simulink model "motor1"  (R2022b)
settings: Solver=ode3  StartTime=0.0  StopTime=10  FixedStep=0.001  MaxStep=0.0001  RelTol=1e-3
undefined symbols (not defined in the file or in its folder): awu, dac, degs2rpm, diff, National_Instruments, PCIe, pid, rpm2rads, sens, step
libraries: sldrtlib x3
settings Model: SimulationMode=external  ExtModeTrigDuration=50000  Creator=loren  LastModifiedBy=francesch2
settings DataIOCC: ReturnWorkspaceOutputs=off
settings HardwareCC: ProdBitPerLong=64  ProdHWDeviceType=Intel->x86-64 (Linux 64)
settings ModelReferenceCC: EnableRefExpFcnMdlSchedulingChecks=on
settings RTWCC: Description=Simulink Desktop Real-Time  SystemTargetFile=sldrt.tlc  TemplateMakefile=sldrt.tmf  RTWCompilerOptimization=on
settings CodeAppCC: MaxIdLength=95
settings SimulinkDesktopRealTimeCC: TargetLibSuffix=_sldrt.a  TargetPreCompLibLocation=C:\Program Files\MATLAB\R2022b\toolbox\sldrt\lib\win64

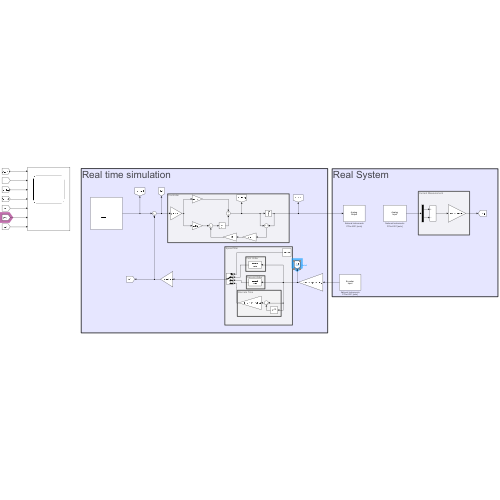
[thumbnail: Simulink's stored preview of the top-level diagram]
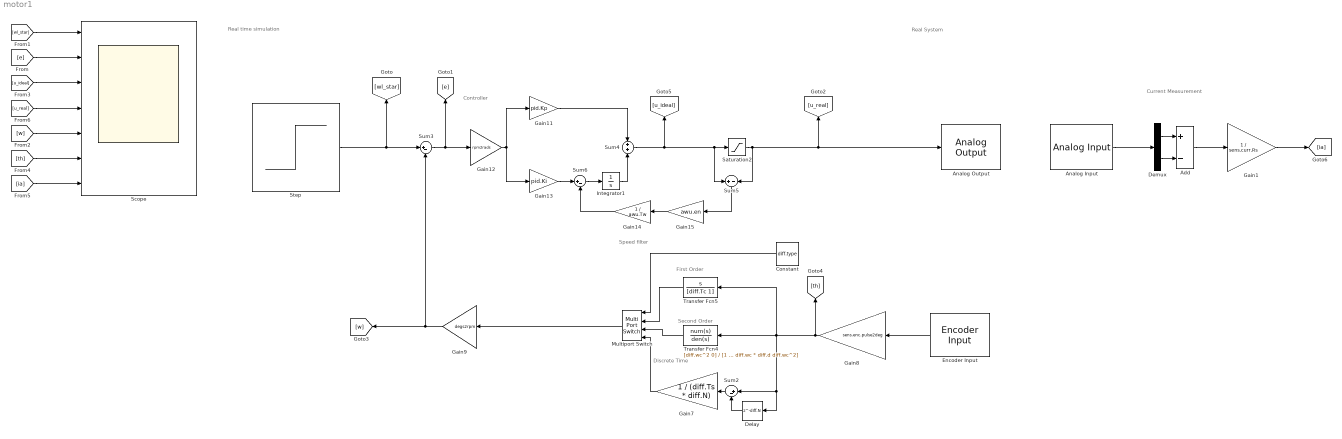
== system motor1 ==
  note: Real time simulation
  note: Controller
  note: Speed filter
  note: Discrete Time
  note: Second Order
  note: First Order
  note: Real System
  note: Current Measurement
  Add : Sum  Inputs=+-
  Analog Input : sldrtlib/Analog Input  SampleTime=-1  MaxMissedTicks=10  ShowMissedTicks=off  YieldWhenWaiting=off  DrvName=National_Instruments/PCIe-6321  DrvAddress=4294967295  DrvOptions=[0 0 0 2 0 0 0]  Channels=[1 2]  RangeMode=1  VoltRange=1  DataType=1
      settings: AttributesFormatString=National Instruments\nPCIe-6321 [auto]
  Analog Output : sldrtlib/Analog Output  SampleTime=-1  MaxMissedTicks=10  ShowMissedTicks=off  YieldWhenWaiting=off  DrvName=National_Instruments/PCIe-6321  DrvAddress=4294967295  DrvOptions=[0 0 0 2 0 0 0]  Channels=1  RangeMode=1  VoltRange=1  InitialValue=0  FinalValue=0
      settings: AttributesFormatString=National Instruments\nPCIe-6321 [auto]
  Constant : Constant  Value=diff.type
  Delay : Delay  DelayLength=diff.N
  Demux : Demux  Outputs=2
  Encoder Input : sldrtlib/Encoder Input  SampleTime=-1  MaxMissedTicks=10  ShowMissedTicks=off  YieldWhenWaiting=off  DrvName=National_Instruments/PCIe-6321  DrvAddress=4294967295  DrvOptions=[0 0 0 2 0 0 0]  Channels=1  QuadMode=3  IndexPulse=1  InputFilter=Inf  DataType=1
      settings: AttributesFormatString=National Instruments\nPCIe-6321 [auto]
  Gain1 : Gain  Gain=1 / sens.curr.Rs
  Gain11 : Gain  Gain=pid.Kp
  Gain12 : Gain  Gain=rpm2rads
  Gain13 : Gain  Gain=pid.Ki
  Gain14 : Gain  Gain=1 / awu.Tw
  Gain15 : Gain  Gain=awu.en
  Gain7 : Gain  Gain=1 / (diff.Ts * diff.N)
  Gain8 : Gain  Gain=sens.enc.pulse2deg
  Gain9 : Gain  Gain=degs2rpm
  Integrator1 : Integrator
  Multiport Switch : MultiPortSwitch  SaturateOnIntegerOverflow=off  InputSameDT=off
  Saturation2 : Saturate  UpperLimit=dac.V  LowerLimit=-dac.V
  Scope : Scope  NumInputPorts=7
  Step : Step  Time=step.T  After=step.A  SampleTime=0
  Sum2 : Sum  Inputs=|+-
  Sum3 : Sum  Inputs=|+-
  Sum4 : Sum  Inputs=+|+
  Sum5 : Sum  Inputs=+|-
  Sum6 : Sum  Inputs=|+-
  Transfer Fcn4 : TransferFcn  Numerator=[diff.wc^2 0]  Denominator=[1 2 * diff.wc * diff.d diff.wc^2]
  Transfer Fcn5 : TransferFcn  Numerator=[1 0]  Denominator=[diff.Tc 1]
  wires:
  Gain8/1 -> Transfer Fcn5/1, Transfer Fcn4/1, Delay/1, Sum2/1, [th]
  Delay/1 -> Sum2/2
  Sum2/1 -> Gain7/1
  Multiport Switch/1 -> Gain9/1
  Transfer Fcn5/1 -> Multiport Switch/2
  Transfer Fcn4/1 -> Multiport Switch/3
  Constant/1 -> Multiport Switch/1
  Gain9/1 -> [w], Sum3/2
  Sum3/1 -> [e], Gain12/1
  Gain12/1 -> Gain11/1, Gain13/1
  Sum4/1 -> Saturation2/1, Sum5/1, [u_ideal]
  Gain11/1 -> Sum4/1
  Integrator1/1 -> Sum4/2
  Gain7/1 -> Multiport Switch/4
  Step/1 -> [wl_star], Sum3/1
  Gain13/1 -> Sum6/1
  Sum6/1 -> Integrator1/1
  Saturation2/1 -> [u_real], Analog Output/1, Sum5/2
  Sum5/1 -> Gain15/1
  Gain14/1 -> Sum6/2
  Gain15/1 -> Gain14/1
  [w] -> Scope/5
  [ia] -> Scope/7
  [wl_star] -> Scope/1
  [u_ideal] -> Scope/3
  [e] -> Scope/2
  Add/1 -> Gain1/1
  Demux/2 -> Add/2
  [th] -> Scope/6
  Gain1/1 -> [ia]
  Demux/1 -> Add/1
  Analog Input/1 -> Demux/1
  Encoder Input/1 -> Gain8/1
  [u_real] -> Scope/4
